simulink model "sim_2309"  (R2023a)
settings: Solver=FixedStepAuto  StartTime=0.0  StopTime=0.03  FixedStep=1e-7  RelTol=1e-3
values from neighbouring files (symbols this model uses):
  J = 83e-6    (= 8.3e-05)    [donnees2309.m]
  kphi = 0.127    [donnees2309.m]
  L = 2.2e-3    (= 0.0022)    [donnees2309.m]
  R = 1.52    [donnees2309.m]
settings Model: Creator=magic  LastModifiedBy=magic

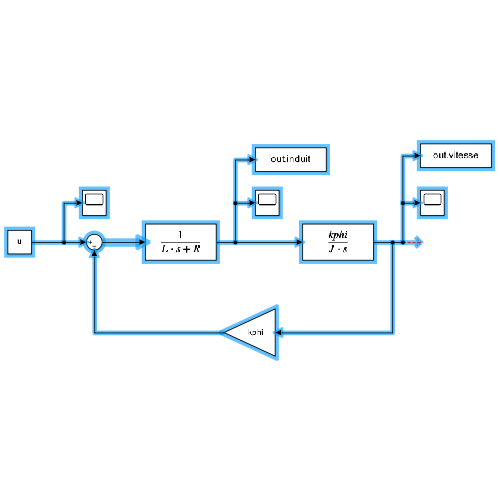
[thumbnail: Simulink's stored preview of the top-level diagram]
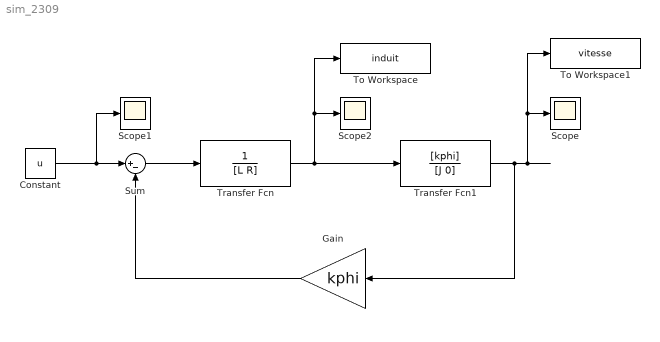
== system sim_2309 ==
  Constant : Constant  Value=u
  Gain : Gain  Gain=kphi
  Scope : Scope
  Scope1 : Scope
  Scope2 : Scope
  Sum : Sum  Inputs=|+-
  To Workspace : ToWorkspace  VariableName=induit  SaveFormat=Timeseries  SampleTime=-1
  To Workspace1 : ToWorkspace  VariableName=vitesse  SaveFormat=Timeseries  SampleTime=-1
  Transfer Fcn : TransferFcn  Denominator=[L R]
  Transfer Fcn1 : TransferFcn  Numerator=[kphi]  Denominator=[J 0]
  wires:
  Constant/1 -> Scope1/1, Sum/1
  Transfer Fcn1/1 -> To Workspace1/1, Scope/1, Gain/1
  Gain/1 -> Sum/2
  Transfer Fcn/1 -> To Workspace/1, Scope2/1, Transfer Fcn1/1
  Sum/1 -> Transfer Fcn/1
